simulink model "CruiseControlModel"  (R2024a)
settings: Solver=ode15s  StartTime=0.0  StopTime=30  RelTol=1e-3  AbsTol=1e-3
values from neighbouring files (symbols this model uses):
  A = 1.4    [CruiseControl.m]
  Ca = 0.3    [CruiseControl.m]
  Ff = mu * Mv * g    (= 117.72)    [CruiseControl.m]
  Fg = Mv * g    (= 11772)    [CruiseControl.m]
  p = 1.225    [CruiseControl.m]
libraries: fl_lib x20, nesl_utility x5, slpidlib x1
settings Model: Creator=macbookair  LastModifiedBy=macbookair
settings SolverCC: AutoScaleAbsTol=off  AlgebraicLoopSolver=TrustRegion  MaxZcPerStep=1
settings DebuggingCC: UnconnectedInputMsg=warning  UnconnectedOutputMsg=warning  UnconnectedLineMsg=warning  SymbolicDimsDataTypeCodeGenerationDiagnostic=none
settings ModelReferenceCC: EnableRefExpFcnMdlSchedulingChecks=on
settings SFSimCC: CustomCodeUndefinedFunction=UseInterfaceOnly
settings RTWCC: GPUComputeCapability=3.5  DLArmComputeVersion=19.05
settings SimscapeCC: SimscapeLogType=all  SimscapeLogSimulationStatistics=on  SimscapeLogDataHistory=10000

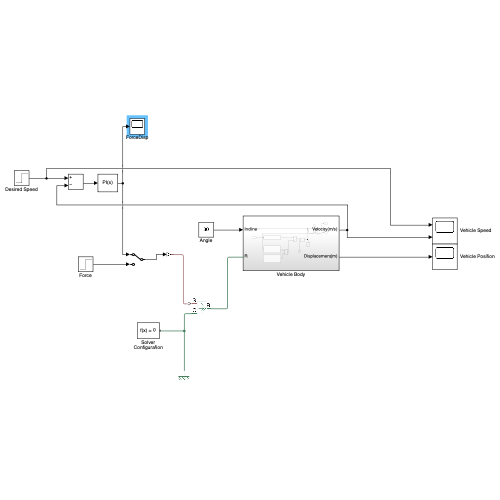
[thumbnail: Simulink's stored preview of the top-level diagram]
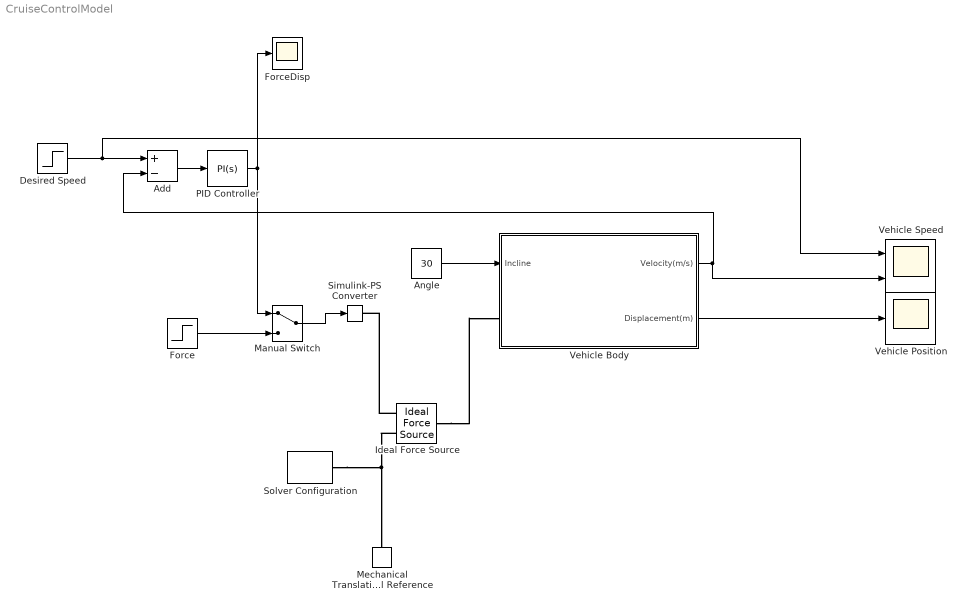
== system CruiseControlModel ==
  Add : Sum  Inputs=+-
  Angle : Constant  Value=30
  Desired Speed : Step  Before=15  After=15  SampleTime=0
  Force : Step  After=7000  SampleTime=0
  ForceDisp : Scope
  Ideal Force Source : fl_lib/Mechanical/Mechanical Sources/Ideal Force Source
  Manual Switch : ManualSwitch
  Mechanical Translational Reference : fl_lib/Mechanical/Translational Elements/Mechanical Translational Reference
  PID Controller : slpidlib/PID Controller  Controller=PI  Form=Parallel  TimeDomain=Continuous-time  UseExternalTs=off  SampleTime=-1  IntegratorMethod=Forward Euler  FilterMethod=Forward Euler  ControllerParametersSource=internal  P=0.1  I=4400  UseKiTs=off  D=0  UseExternalDerivativeSource=off  N=100  UseFilter=on  TunerSelectOption=Transfer Function Based (PID Tuner App)  InitialConditionSource=internal  InitialConditionForIntegrator=0  InitialConditionForFilter=0  DifferentiatorICPrevScaledInput=0  ExternalReset=none  TrackingMode=off  Kt=1  LimitOutput=off  SatLimitsSource=internal  UpperSaturationLimit=inf  LowerSaturationLimit=-inf  LinearizeAsGain=on  AntiWindupMode=none  Kb=1  LimitIntegrator=off  UpperIntegratorSaturationLimit=inf  LowerIntegratorSaturationLimit=-inf  POutMin=[]  POutMax=[]  IOutMin=[]  IOutMax=[]  DOutMin=[]  DOutMax=[]  NOutMin=[]  NOutMax=[]  SumOutMin=[]  SumOutMax=[]  SaturationOutMin=[]  SaturationOutMax=[]  PParamMin=[]  PParamMax=[]  IParamMin=[]  IParamMax=[]  DParamMin=[]  DParamMax=[]  NParamMin=[]  NParamMax=[]  KbParamMin=[]  KbParamMax=[]  KtParamMin=[]  KtParamMax=[]  KbOutMin=[]  KbOutMax=[]  KtOutMin=[]  KtOutMax=[]  IntegratorOutMin=[]  IntegratorOutMax=[]  FilterOutMin=[]  FilterOutMax=[]  SumI1OutMin=[]  SumI1OutMax=[]  SumI2OutMin=[]  SumI2OutMax=[]  SumI3OutMin=[]  SumI3OutMax=[]  SumI4OutMin=[]  SumI4OutMax=[]  SumDOutMin=[]  SumDOutMax=[]  DifferentiatorOutMin=[]  DifferentiatorOutMax=[]  FilterDiffOutCoefMin=[]  FilterDiffOutCoefMax=[]  ReciprocalOutMin=[]  ReciprocalOutMax=[]  SumDenOutMin=[]  SumDenOutMax=[]  SumNumOutMin=[]  SumNumOutMax=[]  DivideOutMin=[]  DivideOutMax=[]  UdiffTsProdOutMin=[]  UdiffTsProdOutMax=[]  NTsProdOutMin=[]  NTsProdOutMax=[]  UintegralTsProdOutMin=[]  UintegralTsProdOutMax=[]  UngainTsProdOutMin=[]  UngainTsProdOutMax=[]  ClampingZeroOutDataTypeStr=Inherit: Inherit via back propagation  ClampingZeroOutMin=[]  ClampingZeroOutMax=[]  FilterDenConstantOutDataTypeStr=Inherit: Inherit via back propagation  FilterDenConstantOutMin=[]  FilterDenConstantOutMax=[]  PCopyOutDataTypeStr=Inherit: Inherit via back propagation  PCopyOutMin=[]  PCopyOutMax=[]  NCopyOutDataTypeStr=Inherit: Inherit via back propagation  NCopyOutMin=[]  NCopyOutMax=[]  IntegratorContinuousStateAttributes=''  IntegratorStateMustResolveToSignalObject=off  IntegratorRTWStateStorageClass=Auto  FilterContinuousStateAttributes=''  FilterStateMustResolveToSignalObject=off  FilterRTWStateStorageClass=Auto  ParallelPVariant=InternalParameters  IdealPVariant=Disabled  IVariant=InternalParameters  DVariant=Disabled  IntegratorVariant=Continuous  SatVariant=Disabled  AWVariant=Passthrough  PCopyVariant=Disabled  TRVariant=Disabled  FdbkBlocksVariant=Forward  IdealPFdbkVariant=Disabled  SatFdbkVariant=Disabled  DerivativeFilterVariant=Disabled  NVariant=Disabled  NCopyVariant=Disabled_SignalSpec  FilterICVariant=Disabled  IntegratorICVariant=InternalICs  ExternalResetVariant=Disabled  TRSumVariant=Passthrough  SumFdbkVariant=Disabled  SumVariant=Sum_PI  TsampFilterVariant=InternalTs  TsampNgainVariant=Passthrough  TsampIntegralVariant=Disabled_SignalSpec  ExternalSaturationOutDataTypeStr=Inherit: Same as second input  DerivativeSourceVariant=Disabled
  Simulink-PS Converter : nesl_utility/Simulink-PS Converter  PhysicalDomain=network_engine_domain  SubClassName=ps_input  LeftPortType=input  RightPortType=output  PseudoPeriodic=off  Frequencies=[]  NoiseDistribution=none  NoiseParameters=[]  Unit=1  AffineConversion=off  FilteringAndDerivatives=provide  SimscapeFilterOrder=1  InputFilterTimeConstant=0.001  UdotUserProvided=0
  Solver Configuration : nesl_utility/Solver Configuration  PhysicalDomain=network_engine_domain  SubClassName=solver  LeftPortType=input  RightPortType=generic  Tones=[]  Harmonics=[]  SimulateNoise=off  Profile=off  UseLocalSampling=off  EnableSwitchedLinearOptims=on  FrequencyDomain=off  UseCCode=off  RelTol=0.001  AbsTol=1e-06  MinStep=1e-09  ToWorkspace=off  RevertToSquareIcSolve=off  NumHomotopyIterations=100  PhasorMode=off  PhasorModeNumHarmonics=1  ConsistencySolver=NEWTON_XTOL_AFTER_FTOL  IndexReductionMethod=DerivativeReplacement  DoDC=off  ResidualTolerance=1e-09  ConsistencyTolSource=GLOBAL  ConsistencyAbsTol=0.001  ConsistencyRelTol=0.001  ConsistencyTolFactor=0.001  UseLocalSolver=off  LocalSolverChoice=NE_BACKWARD_EULER_ADVANCER  ResolveIndetEquations=on  FunctionEvalNumThread=1  LocalSolverSampleTime=0.001  DoFixedCost=off  MaxNonlinIter=3  MaxModeIter=2  ComputeImpulses=off  ImpulseIterations=2  LinearAlgebra=auto  LinearAlgebraNumThread=0  EquationFormulation=NE_TIME_EF  DelaysMemoryBudget=1024  AutomaticFiltering=on  FilteringTimeConstant=0.001  PartitionStorageMethod=AS_NEEDED  PartitionMemoryBudget=1024  PartitionMethod=ROBUST  MultibodyUseLocalSolver=off  MultibodyLocalSolverChoice=ODE1  MultibodyLocalSolverSampleTime=0.001
  Vehicle Body : Subsystem
  Vehicle Position : Scope
  Vehicle Speed : Scope  NumInputPorts=2
  wires:
  Desired Speed/1 -> Vehicle Speed/1, Add/1
  Vehicle Body/1(Velocity(m/s)) -> Vehicle Speed/2, Add/2
  Vehicle Body/2(Displacement(m)) -> Vehicle Position/1
  Add/1 -> PID Controller/1
  Force/1 -> Manual Switch/2
  PID Controller/1 -> Manual Switch/1, ForceDisp/1
  Manual Switch/1 -> Simulink-PS Converter/1
  Angle/1 -> Vehicle Body/1(Incline)
  connections:
  Ideal Force Source/RConn1 -- Simulink-PS Converter/RConn1
  Ideal Force Source/RConn2 -- Solver Configuration/RConn1 -- Mechanical Translational Reference/LConn1
  Ideal Force Source/LConn1 -- Vehicle Body/LConn1

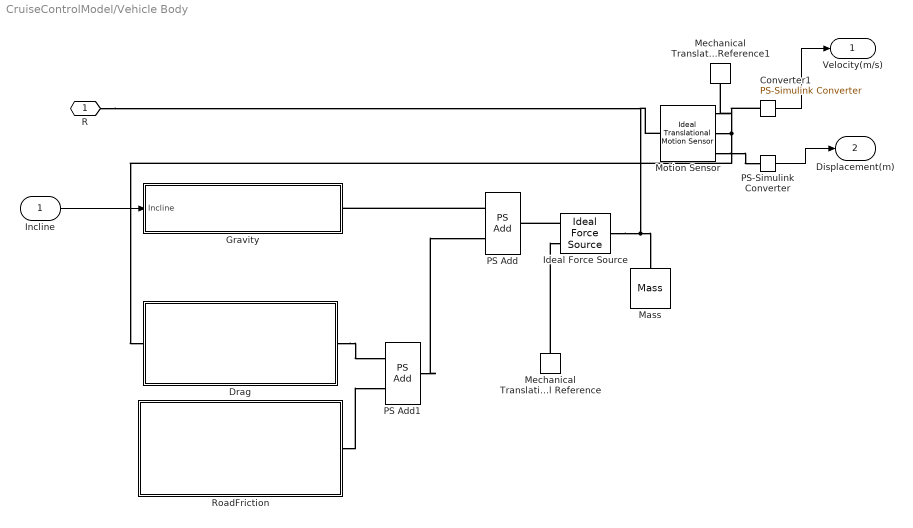
== system CruiseControlModel/Vehicle Body ==
  Incline : Inport
  Converter1 : nesl_utility/PS-Simulink Converter  PhysicalDomain=network_engine_domain  SubClassName=ps_output  LeftPortType=input  RightPortType=output  PseudoPeriodic=off  Frequencies=[]  VectorFormat=inherit  Unit=m/s  AffineConversion=off
  Drag : Subsystem
  Gravity : Subsystem
  Ideal Force Source : fl_lib/Mechanical/Mechanical Sources/Ideal Force Source
  Mass : fl_lib/Mechanical/Translational Elements/Mass  mass=Mv kg  num_ports=foundation.enum.numPorts2.one  v_specify=off  v_priority=High  v=0 m/s  v_nominal_specify=off  v_nominal_value=1  v_nominal_unit=m/s  f_specify=off  f_priority=None  f=0 N  f_nominal_specify=off  f_nominal_value=1  f_nominal_unit=N
  Mechanical Translational Reference : fl_lib/Mechanical/Translational Elements/Mechanical Translational Reference
  Mechanical Translational Reference1 : fl_lib/Mechanical/Translational Elements/Mechanical Translational Reference
  Motion Sensor : fl_lib/Mechanical/Mechanical Sensors/Ideal Translational Motion Sensor  reference=foundation.enum.MeasurementReference.difference  acceleration_port=false  velocity_port=true  position_port=true  offset=0 m
  PS Add : fl_lib/Physical Signals/Functions/PS Add
  PS Add1 : fl_lib/Physical Signals/Functions/PS Add
  PS-Simulink Converter : nesl_utility/PS-Simulink Converter  PhysicalDomain=network_engine_domain  SubClassName=ps_output  LeftPortType=input  RightPortType=output  PseudoPeriodic=off  Frequencies=[]  VectorFormat=inherit  Unit=m  AffineConversion=off
  RoadFriction : Subsystem
  R : PMIOPort  Side=Left
  Velocity(m/s) : Outport
  Displacement(m) : Outport  Port=2
  wires:
  Converter1/1 -> Velocity(m/s)/1
  Incline/1 -> Gravity/1(Incline)
  PS-Simulink Converter/1 -> Displacement(m)/1
  connections:
  PS Add1/RConn1 -- PS Add/LConn2
  Ideal Force Source/LConn1 -- Mass/LConn1 -- Motion Sensor/LConn1 -- R/RConn1
  Motion Sensor/RConn2 -- Drag/LConn1 -- Converter1/LConn1
  Ideal Force Source/RConn1 -- PS Add/RConn1
  Mechanical Translational Reference/LConn1 -- Ideal Force Source/RConn2
  PS Add/LConn1 -- Gravity/RConn1
  Drag/RConn1 -- PS Add1/LConn1
  RoadFriction/RConn1 -- PS Add1/LConn2
  Motion Sensor/RConn3 -- PS-Simulink Converter/LConn1
  Motion Sensor/RConn1 -- Mechanical Translational Reference1/LConn1

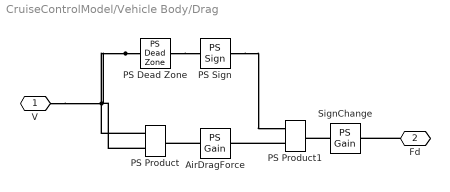
== system CruiseControlModel/Vehicle Body/Drag ==
  AirDragForce : fl_lib/Physical Signals/Functions/PS Gain  gain=0.5 * Ca * A * p
  PS Dead Zone : fl_lib/Physical Signals/Nonlinear Operators/PS Dead Zone  upper_limit=0.5 m/s  lower_limit=-0.5 m/s
      settings: InternalSimscapePortConfiguration="{\"Bottom\":[],\"Left\":[{\"id\":\"I\",\"label\":\"\",\"type\":\"input\"}],\"Right\":[{\"id\":\"O\",\"label\":\"\",\"type\":\"output\"}],\"Top\":[]}"
  PS Product : fl_lib/Physical Signals/Functions/PS Product
  PS Product1 : fl_lib/Physical Signals/Functions/PS Product
  PS Sign : fl_lib/Physical Signals/Nonlinear Operators/PS Sign
      settings: InternalSimscapePortConfiguration="{\"Bottom\":[],\"Left\":[{\"id\":\"I\",\"label\":\"\",\"type\":\"input\"}],\"Right\":[{\"id\":\"O\",\"label\":\"\",\"type\":\"output\"}],\"Top\":[]}"
  SignChange : fl_lib/Physical Signals/Functions/PS Gain  gain=-1 N*(s^2/m^2)
  V : PMIOPort  Side=Left
  Fd : PMIOPort  Port=2  Side=Right
  connections:
  PS Dead Zone/RConn1 -- PS Sign/LConn1
  AirDragForce/LConn1 -- PS Product/RConn1
  PS Sign/RConn1 -- PS Product1/LConn1
  PS Product1/LConn2 -- AirDragForce/RConn1
  SignChange/LConn1 -- PS Product1/RConn1
  PS Dead Zone/LConn1 -- V/RConn1 -- PS Product/LConn2 -- PS Product/LConn1
  Fd/RConn1 -- SignChange/RConn1

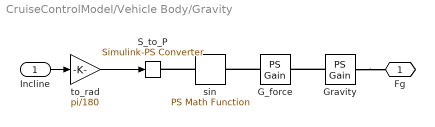
== system CruiseControlModel/Vehicle Body/Gravity ==
  Incline : Inport
  G_force : fl_lib/Physical Signals/Functions/PS Gain  gain=Fg N
  Gravity : fl_lib/Physical Signals/Functions/PS Gain  gain=-1
  S_to_P : nesl_utility/Simulink-PS Converter  PhysicalDomain=network_engine_domain  SubClassName=ps_input  LeftPortType=input  RightPortType=output  PseudoPeriodic=off  Frequencies=[]  NoiseDistribution=none  NoiseParameters=[]  Unit=1  AffineConversion=off  FilteringAndDerivatives=provide  SimscapeFilterOrder=1  InputFilterTimeConstant=0.001  UdotUserProvided=0
  sin : fl_lib/Physical Signals/Functions/PS Math Function  fcn_choice=foundation.enum.math_function.sin  v=1
  to_rad : Gain  Gain=pi/180
  Fg : PMIOPort  Side=Right
  wires:
  Incline/1 -> to_rad/1
  to_rad/1 -> S_to_P/1
  connections:
  sin/LConn1 -- S_to_P/RConn1
  G_force/LConn1 -- sin/RConn1
  Gravity/RConn1 -- Fg/RConn1
  Gravity/LConn1 -- G_force/RConn1

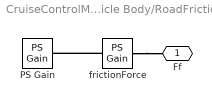
== system CruiseControlModel/Vehicle Body/RoadFriction ==
  PS Gain : fl_lib/Physical Signals/Functions/PS Gain  gain=Ff N
  frictionForce : fl_lib/Physical Signals/Functions/PS Gain  gain=-1
  Ff : PMIOPort  Side=Right
  connections:
  frictionForce/RConn1 -- Ff/RConn1
  frictionForce/LConn1 -- PS Gain/RConn1
